simulink model "Autopilot_q_full_5may_new"  (R2020a)
settings: Solver=ode4  StartTime=0.0  StopTime=300  FixedStep=0.01  RelTol=1e-3
undefined symbols (not defined in the file or in its folder): Aero_cofficients, Atmosphere_pert, Atmospheric_model, Counter_sensor_model, Earth, error_global, flags_global, Guidance_Flags_global, INT_global, param_guidance, Payload_data, Plane_state_mode_finish_catcher_ftr_mode, Plane_state_mode_finish_catcher_fw_mode, Plane_state_mode_finish_catcher_q_mode, Plane_state_mode_finish_catcher_rtr_mode, Plane_state_store, propulsion_model, propulsion_model_int, Structural_data, Thrust_data_store, time_global, WGS84, Wind_data, Wind_model_int, Wind_pert_factor
libraries: simulink x33, aerolibactuator x15, cstblocks x3, aerolibatmos2 x2, aerolibfltsims x1, aerolibtransform2 x1, shared6dof x1
(part 9 of 10)

== matlab function Autopilot_q_full_5may_new/AUTOPILOT /Autopilot Fixed wing mode/Pitch controller/MATLAB Function3 ==
  data: a_z_d input; Plane_state input; aero_data input; structure_data input; alpha_d output; Thrust input; Wind_ned input; propulsion_data input; atmos_data input; data2 input; data3 input; data4 input; data5 input; data6 input; data7 input
function alpha_d = Autopilot(a_z_d,Plane_state, aero_data, structure_data, Thrust, Wind_ned,  propulsion_data, atmos_data, data2, data3, data4, data5, data6, data7)
%%
b1=propulsion_data(1); % b and d of vtol propellers
d1=propulsion_data(2);
b1_inv=1.0/b1;
%%
rho=atmos_data(4); % density
%%
Tzf1=Thrust(1);
Tzf2=Thrust(2);
Tzf3=Thrust(3);
Tzf4=Thrust(4);

Tzb5=Thrust(5);
Tzb6=Thrust(6);
Tzb7=Thrust(7);
Tzb8=Thrust(8);
Tx9=Thrust(9);
Tx10=Thrust(10);
delta_e=Thrust(11);
delta_a=Thrust(12);
delta_r=Thrust(13);


mass=structure_data(1,1);c=structure_data(1,2);b=structure_data(1,3);s=structure_data(1,4);
Ix=structure_data(1,5);Iy=structure_data(1,6);Iz=structure_data(1,7);
Ixy=structure_data(1,8);Ixz=structure_data(1,9);Iyz=structure_data(1,10);
x1=structure_data(1,11);x2=structure_data(1,12);y1=structure_data(1,13);y2=structure_data(1,14);
y3=structure_data(1,15);y4=structure_data(1,16);y5=structure_data(1,17);y6=structure_data(1,18);
y7=structure_data(1,19);y8=structure_data(1,20);y9=structure_data(1,21);y10=structure_data(1,22);
z1=structure_data(1,23);mb=structure_data(1,24);

T_by_W=2.0;

c0=Ix*Iz-Ixz^2;
c1=Ixz*(Ix-Iy+Iz)/c0;
c2=(Iz*(Iz-Iy)+Ixz^2)/c0;
c3=Iz/c0;
c4=Ixz/c0;
c5=(Iz-Ix)/c0;
c6=Ixz/Iy;
c7=((Ix-Iy)*Ix + Ixz^2)/c0;
c8=Ix/c0;
c3_inv=1/c3;
c8_inv=1/c8;

CLo =aero_data(1,1); CL_alpha=aero_data(1,2);CL_beta=aero_data(1,3); CL_delta_e=aero_data(1,4); CL_delta_a=aero_data(1,5); CL_delta_r=aero_data(1,6); CL_p=aero_data(1,7);CL_q=aero_data(1,8);CL_r=aero_data(1,9);

Cdo =aero_data(2,1); Cd_alpha=aero_data(2,2);Cd_beta=aero_data(2,3); Cd_delta_e=aero_data(2,4); Cd_delta_a=aero_data(2,5); Cd_delta_r=aero_data(2,6); Cd_p=aero_data(2,7);Cd_q=aero_data(2,8);Cd_r=aero_data(2,9);

CYo =aero_data(3,1); CY_alpha=aero_data(3,2);CY_beta=aero_data(3,3); CY_delta_e=aero_data(3,4); CY_delta_a=aero_data(3,5); CY_delta_r=aero_data(3,6); CY_p=aero_data(3,7);CY_q=aero_data(3,8);CY_r=aero_data(3,9);

Clo =aero_data(4,1); Cl_alpha=aero_data(4,2);Cl_beta=aero_data(4,3); Cl_delta_e=aero_data(4,4); Cl_delta_a=aero_data(4,5); Cl_delta_r=aero_data(4,6); Cl_p=aero_data(4,7);Cl_q=aero_data(4,8);Cl_r=aero_data(4,9);

Cmo =aero_data(5,1); Cm_alpha=aero_data(5,2);Cm_beta=aero_data(5,3); Cm_delta_e=aero_data(5,4); Cm_delta_a=aero_data(5,5); Cm_delta_r=aero_data(5,6); Cm_p=aero_data(5,7);Cm_q=aero_data(5,8);Cm_r=aero_data(5,9);

Cno =aero_data(6,1); Cn_alpha=aero_data(6,2);Cn_beta=aero_data(6,3); Cn_delta_e=aero_data(6,4); Cn_delta_a=aero_data(6,5); Cn_delta_r=aero_data(6,6); Cn_p=aero_data(6,7);Cn_q=aero_data(6,8);Cn_r=aero_data(6,9);
Cd_brake=0.0;brake=0.0;g=9.81;


u=Plane_state(1);
v=Plane_state(2);
w=Plane_state(3);
p=Plane_state(4);
q=Plane_state(5);
r=Plane_state(6);
phi=Plane_state(7);
theta=Plane_state(8);
psi=Plane_state(9);
X=Plane_state(10);
Y=Plane_state(11);
Z=Plane_state(12);


Tzf=Tzf2+Tzf3;
Tzb=Tzb6+Tzb7;
Tx=Tx9+Tx10;


R_v_v1=[cos(psi) sin(psi) 0; -sin(psi) cos(psi) 0; 0 0 1];
R_v1_v2=[cos(theta) 0 -sin(theta) ;0 1 0; sin(theta) 0 cos(theta)];
R_v2_b=[1 0 0;0 cos(phi) sin(phi) ;0 -sin(phi) cos(phi)];
R_v_b=R_v2_b*R_v1_v2*R_v_v1;



V_wind_bd=R_v_b*[Wind_ned(1);Wind_ned(2);Wind_ned(3)];

ppp = [u-V_wind_bd(1); v; w];
u_r=ppp(1);
v_r=ppp(2);
w_r=ppp(3);

V=sqrt(u_r^2+v_r^2+w_r^2);


if (u_r^2+v_r^2+w_r^2)<=0.01
    alpha=0;
else
    alpha=atan2( w_r, u_r);
end


if norm(u_r) < 10^-3  && norm(v_r) < 10^-3 && norm(w_r) < 10^-3
    beta=0;
else
    beta = asin(v_r/sqrt(u_r^2+v_r^2+w_r^2));
end



R_b_s=[cos(alpha) 0 sin(alpha) ;0 1 0; -sin(alpha) 0 cos(alpha)];
R_s_w=[cos(beta) sin(beta) 0; -sin(beta) cos(beta) 0; 0 0 1];
R_w_b=(R_b_s)'*(R_s_w)';


%u_dot_d=acc_d(1);
%v_dot_d=acc_d(2);
w_dot_d=a_z_d;



mg_b = R_v_b*[0 ;0; mass*g];
D=0.5*rho*V*V*s*(Cdo+Cd_alpha*abs(alpha)+Cd_delta_e*abs(delta_e)+ Cd_brake*abs(brake)) ;
D_b=R_w_b*[-D;0;0];

if V<0.1
    CL = CLo + CL_alpha*alpha + CL_delta_e*delta_e ;
else
    CL = CLo + CL_alpha*alpha + CL_delta_e*delta_e  + CL_q*q*c/(2*V) ;
end
L=0.5*rho*V*V*s*(CL);
%L_b = R_w_b*[0;0;-L];



fz=mass*w_dot_d;


alpha_d = (1.0/CL_alpha)*(((1.0/(-cos(alpha)*0.5*rho*V*V*s))*(fz - mg_b(3) - D_b(3))) - (CLo  + CL_delta_e*delta_e));


if (alpha_d > (10.0/57.3))
    alpha_d = (10.0/57.3);
end

if ((alpha_d) < (-5.0/57.3))
    
    alpha_d = -5.0/57.3;
end

== matlab function Autopilot_q_full_5may_new/AUTOPILOT /Autopilot Fixed wing mode/Roll controller/MATLAB Function1 ==
  data: t input; Thrust input; mass input; a_y_d input; phi_d output; aero_data input; structure_data input; Plane_state input; param_guidance input; Wind_ned input; propulsion_data input; atmos_data input; data2 input; data3 input; data5 input; data4 input; data6 input; data7 input
function phi_d  = fcn(t, Thrust, mass, a_y_d,aero_data, structure_data,Plane_state, param_guidance, Wind_ned, propulsion_data, atmos_data, data2, data3, data5, data4, data6, data7)
%%
b1=propulsion_data(1); % b and d of vtol propellers
d1=propulsion_data(2);
b1_inv=1.0/b1;
%%
rho=atmos_data(4); % density
%%
R_circ=param_guidance(1);
cruise_speed=param_guidance(2);

lmt_pos=param_guidance(3); lmt_vel=param_guidance(4);

Tzf1=Thrust(1);
Tzf2=Thrust(2);
Tzf3=Thrust(3);
Tzf4=Thrust(4);

Tzb5=Thrust(5);
Tzb6=Thrust(6);
Tzb7=Thrust(7);
Tzb8=Thrust(8);
Tx9=Thrust(9);
Tx10=Thrust(10);
delta_e=Thrust(11);
delta_a=Thrust(12);
delta_r=Thrust(13);

TT=abs(Tzf1+Tzf2+Tzf3+Tzf4+Tzb5+Tzb6+Tzb7+Tzb8);

mass=structure_data(1,1);c=structure_data(1,2);b=structure_data(1,3);s=structure_data(1,4);
% Ix=structure_data(1,5);Iy=structure_data(1,6);Iz=structure_data(1,7);
% Ixy=structure_data(1,8);Ixz=structure_data(1,9);Iyz=structure_data(1,10);
% x1=structure_data(1,11);x2=structure_data(1,12);y1=structure_data(1,13);y2=structure_data(1,14);
% y3=structure_data(1,15);y4=structure_data(1,16);y5=structure_data(1,17);y6=structure_data(1,18);
% y7=structure_data(1,19);y8=structure_data(1,20);y9=structure_data(1,21);y10=structure_data(1,22);
% z1=structure_data(1,23);mb=structure_data(1,24);
%
% T_by_W=2.0;

% c0=Ix*Iz-Ixz^2;
% c1=Ixz*(Ix-Iy+Iz)/c0;
% c2=(Iz*(Iz-Iy)+Ixz^2)/c0;
% c3=Iz/c0;
% c4=Ixz/c0;
% c5=(Iz-Ix)/c0;
% c6=Ixz/Iy;
% c7=((Ix-Iy)*Ix + Ixz^2)/c0;
% c8=Ix/c0;
% c3_inv=1/c3;
% c8_inv=1/c8;

CLo =aero_data(1,1); CL_alpha=aero_data(1,2);CL_beta=aero_data(1,3); CL_delta_e=aero_data(1,4); CL_delta_a=aero_data(1,5); CL_delta_r=aero_data(1,6); CL_p=aero_data(1,7);CL_q=aero_data(1,8);CL_r=aero_data(1,9);

% Cdo =aero_data(1,1); Cd_alpha=aero_data(1,2);Cd_beta=aero_data(1,3); Cd_delta_e=aero_data(1,4); Cd_delta_a=aero_data(1,5); Cd_delta_r=aero_data(1,6); Cd_p=aero_data(1,7);Cd_q=aero_data(1,8);Cd_r=aero_data(1,9);
%
% CYo =aero_data(1,1); CY_alpha=aero_data(1,2);CY_beta=aero_data(1,3); CY_delta_e=aero_data(1,4); CY_delta_a=aero_data(1,5); CY_delta_r=aero_data(1,6); CY_p=aero_data(1,7);CY_q=aero_data(1,8);CY_r=aero_data(1,9);
%
% Clo =aero_data(1,1); Cl_alpha=aero_data(1,2);Cl_beta=aero_data(1,3); Cl_delta_e=aero_data(1,4); Cl_delta_a=aero_data(1,5); Cl_delta_r=aero_data(1,6); Cl_p=aero_data(1,7);Cl_q=aero_data(1,8);Cl_r=aero_data(1,9);
%
% Cmo =aero_data(1,1); Cm_alpha=aero_data(1,2);Cm_beta=aero_data(1,3); Cm_delta_e=aero_data(1,4); Cm_delta_a=aero_data(1,5); Cm_delta_r=aero_data(1,6); Cm_p=aero_data(1,7);Cm_q=aero_data(1,8);Cm_r=aero_data(1,9);
%
% Cno =aero_data(1,1); Cn_alpha=aero_data(1,2);Cn_beta=aero_data(1,3); Cn_delta_e=aero_data(1,4); Cn_delta_a=aero_data(1,5); Cn_delta_r=aero_data(1,6); Cn_p=aero_data(1,7);Cn_q=aero_data(1,8);Cn_r=aero_data(1,9);

% Cd_brake=0.0;brake=0.0;g=9.81;
% b1=0.0007488;
% d1=0.00002828;
% b1_inv=1.0/b1;

u=Plane_state(1);
v=Plane_state(2);
w=Plane_state(3);
p=Plane_state(4);
q=Plane_state(5);
r=Plane_state(6);
phi=Plane_state(7);
theta=Plane_state(8);
psi=Plane_state(9);
% X=Plane_state(10);
% Y=Plane_state(11);
% Z=Plane_state(12);


R_v_v1=[cos(psi) sin(psi) 0; -sin(psi) cos(psi) 0; 0 0 1];
R_v1_v2=[cos(theta) 0 -sin(theta) ;0 1 0; sin(theta) 0 cos(theta)];
R_v2_b=[1 0 0;0 cos(phi) sin(phi) ;0 -sin(phi) cos(phi)];
R_v_b=R_v2_b*R_v1_v2*R_v_v1;



V_wind_bd=R_v_b*[Wind_ned(1);Wind_ned(2);Wind_ned(3)];

ppp = [u-V_wind_bd(1); v; w];
u_r=ppp(1);
v_r=ppp(2);
w_r=ppp(3);

V=sqrt(u_r^2+v_r^2+w_r^2);



if (u_r^2+v_r^2+w_r^2)<=0.01
    alpha=0;
else
    alpha=atan2( w_r, u_r);
end

if norm(u_r) < 10^-3  && norm(v_r) < 10^-3 && norm(w_r) < 10^-3
    beta=0;
else
    beta = asin(v_r/sqrt(u_r^2+v_r^2+w_r^2));
end



R_b_s=[cos(alpha) 0 sin(alpha) ;0 1 0; -sin(alpha) 0 cos(alpha)];
R_s_w=[cos(beta) sin(beta) 0; -sin(beta) cos(beta) 0; 0 0 1];
R_w_b=(R_b_s)'*(R_s_w)';

%
% mg_b = R_v_b*[0 ;0; mass*g];
% D=0.5*rho*V*V*s*(Cdo+Cd_alpha*abs(alpha)+Cd_delta_e*abs(delta_e)+ Cd_brake*abs(brake)) ;
% D_b=R_w_b*[-D;0;0];

if V<0.1
    CL = CLo + CL_alpha*alpha + CL_delta_e*delta_e ;
else
    CL = CLo + CL_alpha*alpha + CL_delta_e*delta_e  + CL_q*q*c/(2*V) ;
end

L=0.5*rho*V*V*s*(CL);



%phi_d=asin((mass/(TT-L_b(3)))*a_y_d);


if ((mass*cruise_speed^2/R_circ)/(abs(L))) > 0.5
    phi_d = sign(R_circ)*30/57.3;
else
    phi_d = asin((mass*cruise_speed^2/R_circ)/(abs(L)));
end
if L<(0.8*mass*9.81)
    phi_d=0.0;
end

if abs(phi_d)>30/57.3
    phi_d=sign(phi_d)*30/57.3;
end


end

== matlab function Autopilot_q_full_5may_new/AUTOPILOT /Autopilot Fixed wing mode/Roll controller/MATLAB Function2 ==
  data: angular_state input; phi_dot_d input; p_d output
function p_d  = fcn(angular_state,phi_dot_d)
p=angular_state(1);
q=angular_state(2);
r=angular_state(3);
phi=angular_state(4);
theta=angular_state(5);
psi=angular_state(6);
p_d= phi_dot_d - q*sin(phi)*tan(theta)-r*cos(phi)*tan(theta);

end

== matlab function Autopilot_q_full_5may_new/AUTOPILOT /Autopilot Transition mode/Reverse transition/Pitch Controller/MATLAB Function3 ==
  data: angular_state input; alpha_dot_d input; q_d output
function q_d  = fcn(angular_state,alpha_dot_d)

% p=angular_state(1);
% q=angular_state(2);
% r=angular_state(3);
% phi=angular_state(4);
% theta=angular_state(5);
% psi=angular_state(6);


		
	q_d=(alpha_dot_d );

	


end

== matlab function Autopilot_q_full_5may_new/AUTOPILOT /Autopilot Transition mode/Forward transition/Pitch Controller/alpha controller/MATLAB Function3 ==
  data: acc_d input; Plane_state input; aero_data input; structure_data input; alpha_d output; Thrust input; Wind_ned input; propulsion_data input; atmos_data input; data2 input; data3 input; data4 input; data5 input; data6 input; data7 input
function alpha_d = Autopilot(acc_d,Plane_state, aero_data, structure_data, Thrust, Wind_ned,  propulsion_data, atmos_data,  data2, data3, data4, data5, data6, data7)
%%
b1=propulsion_data(1); % b and d of vtol propellers
d1=propulsion_data(2);
b1_inv=1.0/b1;
%%
rho=atmos_data(4); % density
%%
Tzf1=Thrust(1);
Tzf2=Thrust(2);
Tzf3=Thrust(3);
Tzf4=Thrust(4);

Tzb5=Thrust(5);
Tzb6=Thrust(6);
Tzb7=Thrust(7);
Tzb8=Thrust(8);
Tx9=Thrust(9);
Tx10=Thrust(10);
delta_e=Thrust(11);
delta_a=Thrust(12);
delta_r=Thrust(13);


mass=structure_data(1,1);c=structure_data(1,2);b=structure_data(1,3);s=structure_data(1,4);
Ix=structure_data(1,5);Iy=structure_data(1,6);Iz=structure_data(1,7);
Ixy=structure_data(1,8);Ixz=structure_data(1,9);Iyz=structure_data(1,10);
x1=structure_data(1,11);x2=structure_data(1,12);y1=structure_data(1,13);y2=structure_data(1,14);
y3=structure_data(1,15);y4=structure_data(1,16);y5=structure_data(1,17);y6=structure_data(1,18);
y7=structure_data(1,19);y8=structure_data(1,20);y9=structure_data(1,21);y10=structure_data(1,22);
z1=structure_data(1,23);mb=structure_data(1,24);

T_by_W=2.0;

c0=Ix*Iz-Ixz^2; 
c1=Ixz*(Ix-Iy+Iz)/c0;    
c2=(Iz*(Iz-Iy)+Ixz^2)/c0;                                              
c3=Iz/c0;
c4=Ixz/c0;
c5=(Iz-Ix)/c0;
c6=Ixz/Iy;
c7=((Ix-Iy)*Ix + Ixz^2)/c0;
c8=Ix/c0;
c3_inv=1/c3;
c8_inv=1/c8;

CLo =aero_data(1,1); CL_alpha=aero_data(1,2);CL_beta=aero_data(1,3); CL_delta_e=aero_data(1,4); CL_delta_a=aero_data(1,5); CL_delta_r=aero_data(1,6); CL_p=aero_data(1,7);CL_q=aero_data(1,8);CL_r=aero_data(1,9);

Cdo =aero_data(2,1); Cd_alpha=aero_data(2,2);Cd_beta=aero_data(2,3); Cd_delta_e=aero_data(2,4); Cd_delta_a=aero_data(2,5); Cd_delta_r=aero_data(2,6); Cd_p=aero_data(2,7);Cd_q=aero_data(2,8);Cd_r=aero_data(2,9);

CYo =aero_data(3,1); CY_alpha=aero_data(3,2);CY_beta=aero_data(3,3); CY_delta_e=aero_data(3,4); CY_delta_a=aero_data(3,5); CY_delta_r=aero_data(3,6); CY_p=aero_data(3,7);CY_q=aero_data(3,8);CY_r=aero_data(3,9);

Clo =aero_data(4,1); Cl_alpha=aero_data(4,2);Cl_beta=aero_data(4,3); Cl_delta_e=aero_data(4,4); Cl_delta_a=aero_data(4,5); Cl_delta_r=aero_data(4,6); Cl_p=aero_data(4,7);Cl_q=aero_data(4,8);Cl_r=aero_data(4,9);

Cmo =aero_data(5,1); Cm_alpha=aero_data(5,2);Cm_beta=aero_data(5,3); Cm_delta_e=aero_data(5,4); Cm_delta_a=aero_data(5,5); Cm_delta_r=aero_data(5,6); Cm_p=aero_data(5,7);Cm_q=aero_data(5,8);Cm_r=aero_data(5,9);

Cno =aero_data(6,1); Cn_alpha=aero_data(6,2);Cn_beta=aero_data(6,3); Cn_delta_e=aero_data(6,4); Cn_delta_a=aero_data(6,5); Cn_delta_r=aero_data(6,6); Cn_p=aero_data(6,7);Cn_q=aero_data(6,8);Cn_r=aero_data(6,9);
Cd_brake=0.0;brake=0.0;g=9.81;


u=Plane_state(1);
v=Plane_state(2);
w=Plane_state(3);
p=Plane_state(4);
q=Plane_state(5);
r=Plane_state(6);
phi=Plane_state(7);
theta=Plane_state(8);
psi=Plane_state(9);
X=Plane_state(10);
Y=Plane_state(11);
Z=Plane_state(12);


        Tzf=Tzf2+Tzf3;
        Tzb=Tzb6+Tzb7;
        Tx=Tx9+Tx10;


R_v_v1=[cos(psi) sin(psi) 0; -sin(psi) cos(psi) 0; 0 0 1];
R_v1_v2=[cos(theta) 0 -sin(theta) ;0 1 0; sin(theta) 0 cos(theta)];
R_v2_b=[1 0 0;0 cos(phi) sin(phi) ;0 -sin(phi) cos(phi)];
R_v_b=R_v2_b*R_v1_v2*R_v_v1;



V_wind_bd=R_v_b*[Wind_ned(1);Wind_ned(2);Wind_ned(3)];

ppp = [u-V_wind_bd(1); v; w];
u_r=ppp(1);
v_r=ppp(2);
w_r=ppp(3);

V=sqrt(u_r^2+v_r^2+w_r^2);





if (u_r^2+v_r^2+w_r^2)<=0.01 
    alpha=0;
else
    alpha=atan2( w_r, u_r);
end

if norm(u_r) < 10^-3  && norm(v_r) < 10^-3 && norm(w_r) < 10^-3
    beta=0;
else
    beta = asin(v_r/sqrt(u_r^2+v_r^2+w_r^2));
end



R_b_s=[cos(alpha) 0 sin(alpha) ;0 1 0; -sin(alpha) 0 cos(alpha)]; 
R_s_w=[cos(beta) sin(beta) 0; -sin(beta) cos(beta) 0; 0 0 1];
R_w_b=(R_b_s)'*(R_s_w)';



u_dot_d=acc_d(1);
v_dot_d=acc_d(2);
w_dot_d=acc_d(3);


mg_b = R_v_b*[0 ;0; mass*g];
D=0.5*rho*V*V*s*(Cdo+Cd_alpha*abs(alpha)+Cd_delta_e*abs(delta_e)+ Cd_brake*abs(brake)) ;
D_b=R_w_b*[-D;0;0];

if V<0.1
    CL = CLo + CL_alpha*alpha + CL_delta_e*delta_e ;
else
    CL = CLo + CL_alpha*alpha + CL_delta_e*delta_e  + CL_q*q*c/(2*V) ;
end
L=0.5*rho*V*V*s*(CL);
L_b = R_w_b*[0;0;-L];

    
        fz=mass*w_dot_d;
    
        
        if (abs(cos(alpha)) >0.1)
        alpha_d = (1.0/CL_alpha)*(((1.0/(-cos(alpha)*0.5*rho*V*V*s))*(fz + (Tzf+Tzb) - mg_b(3) - D_b(3))) - (CLo  + CL_delta_e*delta_e)); 
        else
            alpha_d=3.0/57.3;
        end
       % alpha_d=5.0/57.3;
        
        if (alpha_d > (7.0/57.3))
        	alpha_d = (7.0/57.3);
        end

        if ((alpha_d) < (0.0/57.3))
        
        	alpha_d = 0.0/57.3;
        end

== matlab function Autopilot_q_full_5may_new/AUTOPILOT /Autopilot Transition mode/Forward transition/Pitch Controller/MATLAB Function3 ==
  data: alpha_dot_d input; angular_state input; q_d output
function q_d  = fcn(alpha_dot_d,angular_state)

% p=angular_state(1);
% q=angular_state(2);
% r=angular_state(3);
% phi=angular_state(4);
% theta=angular_state(5);
% psi=angular_state(6);


		
	q_d=(alpha_dot_d );

	


end

== matlab function Autopilot_q_full_5may_new/Wind_Model/Subsystem1/MATLAB Function ==
  data: u input; y output; Wind_model_int input; Z input
function y = fcn(u, Wind_model_int, Z)
y=u;
turb_50=Wind_model_int(8);
turb_50_600=Wind_model_int(9);
turb_600=Wind_model_int(10);

if ((turb_50 == 0) && (Z >=-50))
    y=0.0;  
end

if ((turb_50_600 == 0) && (Z >=-600) && (Z <=-50))
    y=0.0;  
end

if ((turb_600 == 0) && (Z <=-600))
    y=0.0;  
end

if Z>0.0
    y=0.0;
end
end

== matlab function Autopilot_q_full_5may_new/AUTOPILOT /Autopilot Transition mode/Reverse transition/Pitch Controller/MATLAB Function4 ==
  data: theta_dot_d input; angular_state input; q_d output
function q_d  = fcn(theta_dot_d,angular_state)

p=angular_state(1);
q=angular_state(2);
r=angular_state(3);
phi=angular_state(4);
theta=angular_state(5);
psi=angular_state(6);

if (abs(phi)>(pi/2.5))
		
	q_d=(theta_dot_d +r*sin(phi));
		
else
		
	q_d=(theta_dot_d +r*sin(phi))/cos(phi);
end

end

== matlab function Autopilot_q_full_5may_new/AUTOPILOT /Autopilot Transition mode/Reverse transition/Autopilot ==
  data: t input; p_dot_d input; q_dot_d input; r_dot_d input; acc_d input; Tzf1 output; Tzf2 output; Tzf3 output; Tzf4 output; Tzb5 output; Tzb6 output; Tzb7 output; Tzb8 output; Tx9 output; Tx10 output; delta_e output; delta_a output; delta_r output; Plane_state input; aero_data input; structure_data input; Thrust input; flags_global input; time_global input; stall_speed input; flags_global output; time_global output; Wind_ned input; propulsion_data input; atmos_data input; wind_pert_factor input; propulsion_pert_factor input; structure_pert_factor input; atmos_pert_factor input; aero_coff_pert_factor input; data7 input; data8 input; data9 input; data10 input; data11 input; data12 input
function [Tzf1,Tzf2,Tzf3,Tzf4,Tzb5,Tzb6,Tzb7,Tzb8,Tx9,Tx10,delta_e,delta_a,delta_r, flags_global,time_global] = Autopilot(t,p_dot_d,q_dot_d,r_dot_d,acc_d,Plane_state, aero_data, structure_data, Thrust,  flags_global,time_global, stall_speed, Wind_ned, propulsion_data, atmos_data, wind_pert_factor, propulsion_pert_factor, structure_pert_factor, atmos_pert_factor, aero_coff_pert_factor, data7, data8, data9, data10, data11, data12)
%%
b1=propulsion_data(1); % b and d of vtol propellers
d1=propulsion_data(2);
b1_inv=1.0/b1;
% b1 = b1*propulsion_pert_factor(1); % adding in perturbation in b and d
% d1 = d1*propulsion_pert_factor(2);
% b1_inv=1.0/b1;
%%
rho=atmos_data(4); % density
% rho = rho*atmos_pert_factor(4); % adding perturbation in density
%%
tf0=time_global(1);
tf1=time_global(2);
tf2=time_global(3);
tf3=time_global(4);
tf4=time_global(5);
tf5=time_global(6);
tf6=time_global(7);
tf7=time_global(8);
tf8=time_global(9);
%%
all_initial_check_ok=flags_global(1);
default_mode=flags_global(2);
quad_mode=flags_global(3);
Transition_mode=flags_global(4);
Fixed_wing_mode=flags_global(5);
fail_safe_mode=flags_global(6);
fail_safe_mode_hover=flags_global(7);
fail_safe_mode_land=flags_global(8);
fail_safe_mode_2=flags_global(9);
flag_initial_lift_off_hover = flags_global(10);
flag_vertical_takeoff = flags_global(11);
flag_hover_mode = flags_global(12);
flag_circle_mode =  flags_global(13);
flag_cruise_mode = flags_global(14);
flag_vertical_landing = flags_global(15);

one_time_initial_lift_off_hover = flags_global(16);
one_time_initial_vertical_takeoff = flags_global(17);
one_time_initial_hover_mode = flags_global(18);
one_time_initial_cruise_mode = flags_global(19);
one_time_initial_circle_mode = flags_global(20);
one_time_initial_vertical_landing = flags_global(21);

flag_brake_mode=flags_global(22);

flag_forward_transition=flags_global(23);
flag_reverse_transition=flags_global(24);

one_time_initial_flag_forward_transition = flags_global(25);
one_time_initial_flag_reverse_transition = flags_global(26);

%%

Tzf1=Thrust(1);
Tzf2=Thrust(2);
Tzf3=Thrust(3);
Tzf4=Thrust(4);

Tzb5=Thrust(5);
Tzb6=Thrust(6);
Tzb7=Thrust(7);
Tzb8=Thrust(8);
Tx9=Thrust(9);
Tx10=Thrust(10);
delta_e=Thrust(11);
delta_a=Thrust(12);
delta_r=Thrust(13);

%%
mass=structure_data(1,1);c=structure_data(1,2);b=structure_data(1,3);s=structure_data(1,4);
Ix=structure_data(1,5);Iy=structure_data(1,6);Iz=structure_data(1,7);
Ixy=structure_data(1,8);Ixz=structure_data(1,9);Iyz=structure_data(1,10);
x1=structure_data(1,11);x2=structure_data(1,12);y1=structure_data(1,13);y2=structure_data(1,14);
y3=structure_data(1,15);y4=structure_data(1,16);y5=structure_data(1,17);y6=structure_data(1,18);
y7=structure_data(1,19);y8=structure_data(1,20);y9=structure_data(1,21);y10=structure_data(1,22);
z9=structure_data(1,23);mb=structure_data(1,24);
z10=-z9;
 %%
% mass=mass*structure_pert_factor(1,1); % perturbation in structure data
% c=c*structure_pert_factor(1,2);b=b*structure_pert_factor(1,3);s=s*structure_pert_factor(1,4);
% Ix=Ix*structure_pert_factor(1,5);Iy=Iy*structure_pert_factor(1,6);Iz=Iz*structure_pert_factor(1,7);
% Ixy=Ixy*structure_pert_factor(1,8);Ixz=Ixz*structure_pert_factor(1,9);Iyz=Iyz*structure_pert_factor(1,10);
% x1=x1*structure_pert_factor(1,11);x2=x2*structure_pert_factor(1,12);
% y1=y1*structure_pert_factor(1,13);y2=y2*structure_pert_factor(1,14);y3=y3*structure_pert_factor(1,15);y4=y4*structure_pert_factor(1,16);
% y5=y5*structure_pert_factor(1,17);y6=y6*structure_pert_factor(1,18);y7=y7*structure_pert_factor(1,19);y8=y8*structure_pert_factor(1,20);
% y9=y9*structure_pert_factor(1,21);y10=y10*structure_pert_factor(1,22);
% z9=z9*structure_pert_factor(1,23);
% mb=mb*structure_pert_factor(1,24);
% z10=-z9;
% %%
T_by_W=2.0;
%%
c0=Ix*Iz-Ixz^2;
c1=Ixz*(Ix-Iy+Iz)/c0;
c2=(Iz*(Iz-Iy)+Ixz^2)/c0;
c3=Iz/c0;
c4=Ixz/c0;
c5=(Iz-Ix)/c0;
c6=Ixz/Iy;
c7=((Ix-Iy)*Ix + Ixz^2)/c0;
c8=Ix/c0;
c3_inv=1/c3;
c8_inv=1/c8;

%%
CLo =aero_data(1,1); CL_alpha=aero_data(1,2);CL_beta=aero_data(1,3); CL_delta_e=aero_data(1,4); CL_delta_a=aero_data(1,5); CL_delta_r=aero_data(1,6); CL_p=aero_data(1,7);CL_q=aero_data(1,8);CL_r=aero_data(1,9);

Cdo =aero_data(2,1); Cd_alpha=aero_data(2,2);Cd_beta=aero_data(2,3); Cd_delta_e=aero_data(2,4); Cd_delta_a=aero_data(2,5); Cd_delta_r=aero_data(2,6); Cd_p=aero_data(2,7);Cd_q=aero_data(2,8);Cd_r=aero_data(2,9);

CYo =aero_data(3,1); CY_alpha=aero_data(3,2);CY_beta=aero_data(3,3); CY_delta_e=aero_data(3,4); CY_delta_a=aero_data(3,5); CY_delta_r=aero_data(3,6); CY_p=aero_data(3,7);CY_q=aero_data(3,8);CY_r=aero_data(3,9);

Clo =aero_data(4,1); Cl_alpha=aero_data(4,2);Cl_beta=aero_data(4,3); Cl_delta_e=aero_data(4,4); Cl_delta_a=aero_data(4,5); Cl_delta_r=aero_data(4,6); Cl_p=aero_data(4,7);Cl_q=aero_data(4,8);Cl_r=aero_data(4,9);

Cmo =aero_data(5,1); Cm_alpha=aero_data(5,2);Cm_beta=aero_data(5,3); Cm_delta_e=aero_data(5,4); Cm_delta_a=aero_data(5,5); Cm_delta_r=aero_data(5,6); Cm_p=aero_data(5,7);Cm_q=aero_data(5,8);Cm_r=aero_data(5,9);

Cno =aero_data(6,1); Cn_alpha=aero_data(6,2);Cn_beta=aero_data(6,3); Cn_delta_e=aero_data(6,4); Cn_delta_a=aero_data(6,5); Cn_delta_r=aero_data(6,6); Cn_p=aero_data(6,7);Cn_q=aero_data(6,8);Cn_r=aero_data(6,9);

%% perturbation in Aero coffecients
% CLo =CLo*aero_coff_pert_factor(1,1); CL_alpha=CL_alpha*aero_coff_pert_factor(1,2);CL_beta=CL_beta*aero_coff_pert_factor(1,3); CL_delta_e=CL_delta_e*aero_coff_pert_factor(1,4); CL_delta_a=CL_delta_a*aero_coff_pert_factor(1,5); CL_delta_r=CL_delta_r*aero_coff_pert_factor(1,6); CL_p=CL_p*aero_coff_pert_factor(1,7);CL_q=CL_q*aero_coff_pert_factor(1,8);CL_r=CL_r*aero_coff_pert_factor(1,9);
% 
% Cdo =Cdo*aero_coff_pert_factor(2,1); Cd_alpha=Cd_alpha*aero_coff_pert_factor(2,2);Cd_beta=Cd_beta*aero_coff_pert_factor(2,3); Cd_delta_e=Cd_delta_e*aero_coff_pert_factor(2,4); Cd_delta_a=Cd_delta_a*aero_coff_pert_factor(2,5); Cd_delta_r=Cd_delta_r*aero_coff_pert_factor(2,6); Cd_p=Cd_p*aero_coff_pert_factor(2,7);Cd_q=Cd_q*aero_coff_pert_factor(2,8);Cd_r=Cd_r*aero_coff_pert_factor(2,9);
% 
% CYo =CYo*aero_coff_pert_factor(3,1); CY_alpha=CY_alpha*aero_coff_pert_factor(3,2);CY_beta=CY_beta*aero_coff_pert_factor(3,3); CY_delta_e=CY_delta_e*aero_coff_pert_factor(3,4); CY_delta_a=CY_delta_a*aero_coff_pert_factor(3,5); CY_delta_r=CY_delta_r*aero_coff_pert_factor(3,6); CY_p=CY_p*aero_coff_pert_factor(3,7);CY_q=CY_q*aero_coff_pert_factor(3,8);CY_r=CY_r*aero_coff_pert_factor(3,9);
% 
% Clo =Clo*aero_coff_pert_factor(4,1); Cl_alpha=Cl_alpha*aero_coff_pert_factor(4,2);Cl_beta=Cl_beta*aero_coff_pert_factor(4,3); Cl_delta_e=Cl_delta_e*aero_coff_pert_factor(4,4); Cl_delta_a=Cl_delta_a*aero_coff_pert_factor(4,5); Cl_delta_r=Cl_delta_r*aero_coff_pert_factor(4,6); Cl_p=Cl_p*aero_coff_pert_factor(4,7);Cl_q=Cl_q*aero_coff_pert_factor(4,8);Cl_r=Cl_r*aero_coff_pert_factor(4,9);
% 
% Cmo =Cmo*aero_coff_pert_factor(5,1); Cm_alpha=Cm_alpha*aero_coff_pert_factor(5,2);Cm_beta=Cm_beta*aero_coff_pert_factor(5,3); Cm_delta_e=Cm_delta_e*aero_coff_pert_factor(5,4); Cm_delta_a=Cm_delta_a*aero_coff_pert_factor(5,5); Cm_delta_r=Cm_delta_r*aero_coff_pert_factor(5,6); Cm_p=Cm_p*aero_coff_pert_factor(5,7);Cm_q=Cm_q*aero_coff_pert_factor(5,8);Cm_r=Cm_r*aero_coff_pert_factor(5,9);
% 
% Cno =Cno*aero_coff_pert_factor(6,1); Cn_alpha=Cn_alpha*aero_coff_pert_factor(6,2);Cn_beta=Cn_beta*aero_coff_pert_factor(6,3); Cn_delta_e=Cn_delta_e*aero_coff_pert_factor(6,4); Cn_delta_a=Cn_delta_a*aero_coff_pert_factor(6,5); Cn_delta_r=Cn_delta_r*aero_coff_pert_factor(6,6); Cn_p=Cn_p*aero_coff_pert_factor(6,7);Cn_q=Cn_q*aero_coff_pert_factor(6,8);Cn_r=Cn_r*aero_coff_pert_factor(6,9);
%%
Cd_brake=0.0;brake=0.0;g=9.81;
%%
u=Plane_state(1);
v=Plane_state(2);
w=Plane_state(3);
p=Plane_state(4);
q=Plane_state(5);
r=Plane_state(6);
phi=Plane_state(7);
theta=Plane_state(8);
psi=Plane_state(9);
X=Plane_state(10);
Y=Plane_state(11);
Z=Plane_state(12);
%%
Tzf=Tzf2+Tzf3;
Tzb=Tzb6+Tzb7;
Tx=Tx9+Tx10;
%%

R_v_v1=[cos(psi) sin(psi) 0; -sin(psi) cos(psi) 0; 0 0 1];
R_v1_v2=[cos(theta) 0 -sin(theta) ;0 1 0; sin(theta) 0 cos(theta)];
R_v2_b=[1 0 0;0 cos(phi) sin(phi) ;0 -sin(phi) cos(phi)];
R_v_b=R_v2_b*R_v1_v2*R_v_v1;

%%
% 
% Wind_ned(1)=Wind_ned(1)*wind_pert_factor(1);% adding perturbation to wind components
% Wind_ned(2)=Wind_ned(2)*wind_pert_factor(2);
% Wind_ned(3)=Wind_ned(3)*wind_pert_factor(3);

V_wind_bd=R_v_b*[Wind_ned(1);Wind_ned(2);Wind_ned(3)];

ppp = [u-V_wind_bd(1); v; w];
u_r=ppp(1);
v_r=ppp(2);
w_r=ppp(3);

V=sqrt(u_r^2+v_r^2+w_r^2);

%%

if (u_r^2+v_r^2+w_r^2)<=0.01
    alpha=0;
else
    alpha=atan2( w_r, u_r);
end


if norm(u_r) < 10^-3  && norm(v_r) < 10^-3 && norm(w_r) < 10^-3
    beta=0;
else
    beta = asin(v_r/sqrt(u_r^2+v_r^2+w_r^2));
end

%%

R_b_s=[cos(alpha) 0 sin(alpha) ;0 1 0; -sin(alpha) 0 cos(alpha)];
R_s_w=[cos(beta) sin(beta) 0; -sin(beta) cos(beta) 0; 0 0 1];
R_w_b=(R_b_s)'*(R_s_w)';
%%
u_dot_d=acc_d(1);
v_dot_d=acc_d(2);
w_dot_d=acc_d(3);
%%
mg_b = R_v_b*[0 ;0; mass*g];
D=0.5*rho*V*V*s*(Cdo+Cd_alpha*abs(alpha)+Cd_delta_e*abs(delta_e)+ Cd_brake*abs(brake)) ;
D_b=R_w_b*[-D;0;0];

if V<0.1
    CL = CLo + CL_alpha*alpha + CL_delta_e*delta_e ;
else
    CL = CLo + CL_alpha*alpha + CL_delta_e*delta_e  + CL_q*q*c/(2*V) ;
end
L=0.5*rho*V*V*s*(CL);
L_b = R_w_b*[0;0;-L];
if abs(V)<0.1
    CY=CYo + CY_delta_r*delta_r + CY_beta*beta;
else
    CY=CYo + CY_delta_r*delta_r + CY_beta*beta + CY_r*r*b/(2*V);
end
FY=0.5*rho*V*V*s*(CY);
%%
w1=(mass*0.99*g- 0.5*rho*V*V*s*CL)/(0.99*mass*g);
w2=1-w1;
w3=1;
if w1<0.0
    w1=0.0;
    w2=1;
    w3=1;
end

if (u_r<(stall_speed)/2)
    w1=1.0;
    w2=0.0;
    w3=1.0;
end

%%


% if w1<0.05
%
% w1=0.0;
% w2=1.0;
% w3=1.0;
%
%
% Fixed_wing_mode=1;
% Transition_mode=0;
%
% tf4=t;
% end



l_aero=0.5*rho*V^2*s*b*( Clo + Cl_delta_a*delta_a +Cl_delta_r*delta_r +Cl_beta*beta )+0.5*rho*V*s*b*(Cl_p*p*b/2+Cl_r*r*b/2);
m_aero=0.5*rho*V^2*s*c*( Cmo + Cm_alpha*alpha + Cm_delta_e*delta_e)+0.5*rho*V*s*c*Cm_q*q*c/2;
n_aero=0.5*rho*V^2*s*b*( Cno + Cn_delta_a*delta_a +Cn_delta_r*delta_r +Cn_beta*beta )+0.5*rho*V*s*b*(Cn_r*r*b/2+ Cn_p*p*b/2);


l=l_aero...
    + (d1*Tx9*b1_inv) + (d1*Tx10*b1_inv)...
    + (- Tzf2*y2*cos(mb) - Tzf3*y3*cos(mb)   - Tzb6*y6*cos(mb) - Tzb7*y7*cos(mb))...
    + (- Tzf1*y1*cos(mb) - Tzf4*y4*cos(mb)   - Tzb5*y5*cos(mb) - Tzb8*y8*cos(mb));


m=m_aero ...
    + Tx9*z9 + Tx10*z10...
    + Tzf*x1*cos(mb) + Tzb*x2*cos(mb)...
    + d1*Tzf2*b1_inv*sin(mb) - d1*Tzf3*b1_inv*sin(mb) - d1*Tzb6*b1_inv*sin(mb) + d1*Tzb7*b1_inv*sin(mb)...
    + d1*Tzf1*b1_inv*sin(mb) - d1*Tzf4*b1_inv*sin(mb) - d1*Tzb5*b1_inv*sin(mb) + d1*Tzb8*b1_inv*sin(mb);

n=n_aero ...
    - Tx9*y9 - Tx10*y10 ...
    + (Tzf2*x1*sin(mb) - Tzf3*x1*sin(mb) +  Tzb6*x2*sin(mb) - Tzb7*x2*sin(mb))...
    + (Tzf1*x1*sin(mb) - Tzf4*x1*sin(mb) +  Tzb5*x2*sin(mb) - Tzb8*x2*sin(mb))...
    + (- d1*Tzf2*b1_inv*cos(mb) + d1*Tzf3*b1_inv*cos(mb)  + d1*Tzb6*b1_inv*cos(mb)  - d1*Tzb7*b1_inv*cos(mb))...
    + (- d1*Tzf1*b1_inv*cos(mb) + d1*Tzf4*b1_inv*cos(mb)  + d1*Tzb5*b1_inv*cos(mb)  - d1*Tzb8*b1_inv*cos(mb)) ;



% 	fx = Tx9 + Tx10 + D_b(1)+ mg_b(1)+L_b(1);
% 	%%%%%%%%%%%%%%%%%%%%%%%%%%%%%%%%%%%%%%%%%%%%%%%%%%%%%%%%%%%%%%%%%%%%%%%%%%%
% 	fy = (Tzf2*sin(mb) - Tzf3*sin(mb) + Tzb6*sin(mb) - Tzb7*sin(mb)) + D_b(2) + mg_b(2) + FY + L_b(2);
% 	%%%%%%%%%%%%%%%%%%%%%%%%%%%%%%%%%%%%%%%%%%%%%%%%%%%%%%%%%%%%%%%%%%%%%%%%%%%
% 	fz = -Tzf*cos(mb) - Tzb*cos(mb) + mg_b(3)+D_b(3)+L_b(3);
%
%
fx=mass*u_dot_d;
fy=mass*v_dot_d;
fz=mass*w_dot_d;

tam=[-b1*y2,-b1*y3,-b1*y6,-b1*y7; b1*x1,b1*x1,b1*x2,b1*x2; -d1,d1,d1,-d1; -b1,-b1,-b1,-b1];
tbm=zeros(4,1);

tbm(1)=(((p_dot_d - c1*p*q + c2*(q*r) -c4*n)*c3_inv) - l_aero)*w1;%//(((p_dot_d - c1*p*q + c2*(q*r) -c4*n)/c3) - l_aero)*w1*3/8
tbm(2)=(((q_dot_d - c5*p*r + c6*(p*p-r*r))*Iy) - m_aero)*w1;%//(((q_dot_d - c5*p*r + c6*(p*p-r*r))*Iy) - m_aero)*w1/2
tbm(3)=(((r_dot_d - c7*p*q + c1*(q*r) -c4*l)*c8_inv) - n_aero)*w1;%//(((r_dot_d - c7*p*q + c1*(q*r) -c4*l)/c8) - n_aero)*w1/2
tbm(4)=(fz - mg_b(3) - D_b(3) -L_b(3))*w3;%//(mass*w_dot_d - mg_b(3) - D_b(3) -L_b(3))/2

omega_velocity=inv(tam)*tbm;

for i=1:4
    if omega_velocity(i)<0.0
        omega_velocity(i)=0.0;
    end
end
omega_2=sqrt(omega_velocity(1));
omega_3=sqrt(omega_velocity(2));
omega_6=sqrt(omega_velocity(3));
omega_7=sqrt(omega_velocity(4));


Tzf2=b1*omega_2^2;

Tzf3=b1*omega_3^2;

Tzb6=b1*omega_6^2;

Tzb7=b1*omega_7^2;



% tam=[-b1*y1,-b1*y4,-b1*y5,-b1*y8; b1*x1,b1*x1,b1*x2,b1*x2; -d1,d1,d1,-d1; -b1,-b1,-b1,-b1];
% tbm=zeros(4,1);
%
% tbm(1)=(((p_dot_d - c1*p*q + c2*(q*r) -c4*n)*c3_inv) - l_aero)*w1;%//(((p_dot_d - c1*p*q + c2*(q*r) -c4*n)/c3) - l_aero)*w1*3/8
% tbm(2)=(((q_dot_d - c5*p*r + c6*(p*p-r*r))*Iy) - m_aero)*w1;%//(((q_dot_d - c5*p*r + c6*(p*p-r*r))*Iy) - m_aero)*w1/2
% tbm(3)=(((r_dot_d - c7*p*q + c1*(q*r) -c4*l)*c8_inv) - n_aero)*w1;%//(((r_dot_d - c7*p*q + c1*(q*r) -c4*l)/c8) - n_aero)*w1/2
% tbm(4)=(fz - mg_b(3) - D_b(3) -L_b(3))*w3;%//(mass*w_dot_d - mg_b(3) - D_b(3) -L_b(3))/2
%
% omega_velocity=inv(tam)*tbm;
%
% for i=1:4
%     if omega_velocity(i)<0.0
%         omega_velocity(i)=0.0;
%     end
% end
% omega_1=sqrt(omega_velocity(1));
% omega_4=sqrt(omega_velocity(2));
% omega_5=sqrt(omega_velocity(3));
% omega_8=sqrt(omega_velocity(4));
%
%
% Tzf1=b1*omega_1^2;
%
% Tzf4=b1*omega_4^2;
%
% Tzb5=b1*omega_5^2;
%
% Tzb8=b1*omega_8^2;
%

Tzf1=0.0;
Tzf4=0.0;
Tzb5=0.0;
Tzb8=0.0;
Tx10=0.0;

Tx9= fx - (D_b(1)+ mg_b(1)+L_b(1));

Tx9=0.0;

Tzf=Tzf2+Tzf3 + Tzf1 + Tzf4;
Tzb=Tzb6+Tzb7 + Tzb5 + Tzb8;
Tx=Tx9+Tx10;


if (u_r<(stall_speed)/2)
    delta_e=0.0;
    delta_r=0.0;
    delta_a=0.0;
else
    delta_e = (1.0/Cm_delta_e)*(((w2*Iy/(0.5*rho*V*V*s*c))*(q_dot_d - c5*p*r + c6*(p*p-r*r) -((0.0*1.0/Iy)*(Tzf*x1 + Tzb*x2 + Tx9*z9)) )) - (Cmo + Cm_alpha*alpha + (Cm_q*q*c/(2.0*V)))) ;
    delta_a =  (((w2/(0.5*rho*V*V*s*b*c3))*(p_dot_d - c1*p*q + c2*q*r - c4*n))  - (Clo + Cl_beta*beta + Cl_delta_r*delta_r + Cl_r*r*b/(2.0*V) +(Cl_p*p*b/(2.0*V))))/(Cl_delta_a);
    delta_r =  (((w2/(0.5*rho*V*V*s*b*c8))*(r_dot_d - c7*p*q + c1*q*r - c4*l))  - (Cno + Cn_beta*beta + Cn_delta_a*delta_a + Cn_r*r*b/(2.0*V) +(Cn_p*p*b/(2.0*V))))/(Cn_delta_r);
end



if abs(delta_e)>(20.0/57.3)
    delta_e=sign(delta_e)*(20.0/57.3);
end

if abs(delta_a)>(20.0/57.3)
    delta_a=sign(delta_a)*(20.0/57.3);
end

if abs(delta_r)>(20.0/57.3)
    delta_r=sign(delta_r)*(20.0/57.3);
end





if (Tzf > (T_by_W*mass*g)/2.0)
    
    Tzf=(T_by_W*mass*g)/2.0;
end



if(Tzf<= 0.0)
    
    Tzf=0.0;
end

if(Tzb> (T_by_W*mass*g)/2.0)
    
    Tzb=(T_by_W*mass*g)/2.0;
end
if(Tzb<= 0.0)
    
    Tzb=0.0;
end


if(Tzf2<=0.0)
    
    Tzf2=0.0;
end
if(Tzf3<= 0.0)
    
    Tzf3=0.0;
end
if(Tzb6<= 0.0)
    
    Tzb6=0.0;
end
if(Tzb7<=0.0)
    
    Tzb7=0.0;
end
if(Tzf1<=0.0)
    
    Tzf1=0.0;
end
if(Tzf4<= 0.0)
    
    Tzf4=0.0;
end
if(Tzb5<= 0.0)
    
    Tzb5=0.0;
end
if(Tzb8<=0.0)
    
    Tzb8=0.0;
end

if(Tx>120.0)
    
    Tx=120.0;
end

if(Tx< 0.0)
    Tx=0.0;
end

if((Tx9)>120.0)
    Tx9=120.0;
end

if(Tx9 < 0.0)
    Tx9=0.0;
end

if((Tx10)>120.0)
    Tx10=120.0;
end

if(Tx10 < 0.0)
    Tx10=0.0;
end

if(Tzf2>(T_by_W*mass*g)/4.0)
    
    Tzf2 =(T_by_W*mass*g)/4.0;
end

if(Tzf3>=(T_by_W*mass*g)/4.0)
    
    Tzf3 =(T_by_W*mass*g)/4.0;
end

if(Tzb6>=(T_by_W*mass*g)/4.0)
    
    Tzb6 =(T_by_W*mass*g)/4.0;
end

if(Tzb7>=(T_by_W*mass*g)/4.0)
    
    Tzb7 =(T_by_W*mass*g)/4.0;
end


if(Tzf1>(T_by_W*mass*g)/4.0)
    
    Tzf1 =(T_by_W*mass*g)/4.0;
end

if(Tzf4>=(T_by_W*mass*g)/4.0)
    
    Tzf4 =(T_by_W*mass*g)/4.0;
end

if(Tzb5>=(T_by_W*mass*g)/4.0)
    
    Tzb5 =(T_by_W*mass*g)/4.0;
end

if(Tzb8>=(T_by_W*mass*g)/4.0)
    
    Tzb8 =(T_by_W*mass*g)/4.0;
end



flags_global(1)=all_initial_check_ok;
flags_global(2)=default_mode;

flags_global(3)=quad_mode;
flags_global(4)=Transition_mode;
flags_global(5)=Fixed_wing_mode;

flags_global(6)=fail_safe_mode;
flags_global(7)=fail_safe_mode_hover;
flags_global(8)=fail_safe_mode_land;
flags_global(9)=fail_safe_mode_2;


flags_global(10)=flag_initial_lift_off_hover;
flags_global(11)=flag_vertical_takeoff;
flags_global(12)=flag_hover_mode;

flags_global(13)=flag_circle_mode;
flags_global(14)=flag_cruise_mode;

flags_global(15)=flag_vertical_landing;

flags_global(16)=one_time_initial_lift_off_hover;
flags_global(17)=one_time_initial_vertical_takeoff;
flags_global(18)=one_time_initial_hover_mode;
flags_global(19)=one_time_initial_cruise_mode;

flags_global(20)=one_time_initial_circle_mode;
flags_global(21)=one_time_initial_vertical_landing;
flags_global(22)=flag_brake_mode;

flags_global(23)=flag_forward_transition;
flags_global(24)=flag_reverse_transition;
flags_global(25)=one_time_initial_flag_forward_transition;
flags_global(26)=one_time_initial_flag_reverse_transition ;



time_global(1)=tf0;
time_global(2)=tf1;
time_global(3)=tf2;
time_global(4)=tf3;
time_global(5)=tf4;
time_global(6)=tf5;
time_global(7)=tf6;
time_global(8)=tf7;
time_global(9)=tf8;






end

== matlab function Autopilot_q_full_5may_new/AUTOPILOT /Autopilot Transition mode/Reverse transition/MATLAB Function7 ==
  data: v_dot_d output; Plane_state input; data input; acc_d input; u_dot_d output; w_dot_d output; V output
function [v_dot_d,u_dot_d,w_dot_d,V] = fcn(Plane_state, data, acc_d)

u=Plane_state(1);
v=Plane_state(2);
w=Plane_state(3);



V=sqrt(u^2 + v^2 + w^2);

u_dot_d=acc_d(1);
v_dot_d=acc_d(2);
w_dot_d=acc_d(3);

end

== matlab function Autopilot_q_full_5may_new/AUTOPILOT /Autopilot Transition mode/Reverse transition/Trim setting/MATLAB Function ==
  data: aero_data input; structure_data input; V_trim input; alpha_trim output; beta_trim output; delta_e_trim output; delta_a_trim output; delta_r_trim output; Tx_trim output; stall_speed output; propulsion_data input; atmos_data input
function [alpha_trim,beta_trim,delta_e_trim,delta_a_trim,delta_r_trim,Tx_trim,stall_speed]= Autopilot(aero_data,structure_data,V_trim,propulsion_data, atmos_data)
b1=propulsion_data(1); % b and d of vtol propellers
d1=propulsion_data(2);
b1_inv=1.0/b1;
%%
rho=atmos_data(4); % density
%%
V=V_trim;
mass=structure_data(1,1);s=structure_data(1,4);

CLo =aero_data(1,1); CL_alpha=aero_data(1,2);CL_beta=aero_data(1,3); CL_delta_e=aero_data(1,4); CL_delta_a=aero_data(1,5); CL_delta_r=aero_data(1,6); CL_p=aero_data(1,7);CL_q=aero_data(1,8);CL_r=aero_data(1,9);

Cdo =aero_data(2,1); Cd_alpha=aero_data(2,2);Cd_beta=aero_data(2,3); Cd_delta_e=aero_data(2,4); Cd_delta_a=aero_data(2,5); Cd_delta_r=aero_data(2,6); Cd_p=aero_data(2,7);Cd_q=aero_data(2,8);Cd_r=aero_data(2,9);

CYo =aero_data(3,1); CY_alpha=aero_data(3,2);CY_beta=aero_data(3,3); CY_delta_e=aero_data(3,4); CY_delta_a=aero_data(3,5); CY_delta_r=aero_data(3,6); CY_p=aero_data(3,7);CY_q=aero_data(3,8);CY_r=aero_data(3,9);

Clo =aero_data(4,1); Cl_alpha=aero_data(4,2);Cl_beta=aero_data(4,3); Cl_delta_e=aero_data(4,4); Cl_delta_a=aero_data(4,5); Cl_delta_r=aero_data(4,6); Cl_p=aero_data(4,7);Cl_q=aero_data(4,8);Cl_r=aero_data(4,9);

Cmo =aero_data(5,1); Cm_alpha=aero_data(5,2);Cm_beta=aero_data(5,3); Cm_delta_e=aero_data(5,4); Cm_delta_a=aero_data(5,5); Cm_delta_r=aero_data(5,6); Cm_p=aero_data(5,7);Cm_q=aero_data(5,8);Cm_r=aero_data(5,9);

Cno =aero_data(6,1); Cn_alpha=aero_data(6,2);Cn_beta=aero_data(6,3); Cn_delta_e=aero_data(6,4); Cn_delta_a=aero_data(6,5); Cn_delta_r=aero_data(6,6); Cn_p=aero_data(6,7);Cn_q=aero_data(6,8);Cn_r=aero_data(6,9);



g=9.81;



tb=[(mass*g/(0.5*rho*V*V*s)) - CLo;-Cmo];
ta=[CL_alpha,CL_delta_e;Cm_alpha,Cm_delta_e];

trim_set_long = inv(ta)*tb;

alpha_trim = trim_set_long(1);
delta_e_trim = trim_set_long(2);

% CYo + CY_beta*beta + CY_delta_a*delta_a + CY_delta_r*delta_r;
% Clo + Cl_beta*beta + Cl_delta_a*delta_a + Cl_delta_r*delta_r;
% Cno + Cn_beta*beta + Cn_delta_a*delta_a + Cn_delta_r*delta_r;

tb1=[-CYo;-Clo;-Cno];
ta1=[CY_beta,CY_delta_a,CY_delta_r;Cl_beta,Cl_delta_a,Cl_delta_r;Cn_beta,Cn_delta_a,Cn_delta_r];

trim_set_lat=inv(ta1)*tb1;

beta_trim = trim_set_lat(1);
delta_a_trim = trim_set_lat(2);
delta_r_trim = trim_set_lat(3);


% drag = 1/2 *rho *V*V*s*( Cdo + Cd_alpha*alpha + Cd_delta_e*delta_e );
Tx_trim =  0.5*rho*V*V*s*( Cdo + Cd_alpha*alpha_trim + Cd_delta_e*delta_e_trim );

stall_speed=sqrt((mass*g)/(0.5*1.225*s*(CLo+CL_alpha*(12.0/57.3))));

== matlab function Autopilot_q_full_5may_new/AUTOPILOT /Autopilot Transition mode/Reverse transition/Pitch Controller/alpha controller/MATLAB Function3 ==
  data: acc_d input; Plane_state input; aero_data input; structure_data input; alpha_d output; Thrust input; Wind_ned input; propulsion_data input; atmos_data input; data2 input; data3 input; data4 input; data5 input; data6 input; data7 input
function alpha_d = Autopilot(acc_d,Plane_state, aero_data, structure_data, Thrust, Wind_ned, propulsion_data, atmos_data, data2, data3, data4, data5, data6, data7)
%%
b1=propulsion_data(1); % b and d of vtol propellers
d1=propulsion_data(2);
b1_inv=1.0/b1;
%%
rho=atmos_data(4); % density
%%
Tzf1=Thrust(1);
Tzf2=Thrust(2);
Tzf3=Thrust(3);
Tzf4=Thrust(4);

Tzb5=Thrust(5);
Tzb6=Thrust(6);
Tzb7=Thrust(7);
Tzb8=Thrust(8);
Tx9=Thrust(9);
Tx10=Thrust(10);
delta_e=Thrust(11);
delta_a=Thrust(12);
delta_r=Thrust(13);


mass=structure_data(1,1);c=structure_data(1,2);b=structure_data(1,3);s=structure_data(1,4);
Ix=structure_data(1,5);Iy=structure_data(1,6);Iz=structure_data(1,7);
Ixy=structure_data(1,8);Ixz=structure_data(1,9);Iyz=structure_data(1,10);
x1=structure_data(1,11);x2=structure_data(1,12);y1=structure_data(1,13);y2=structure_data(1,14);
y3=structure_data(1,15);y4=structure_data(1,16);y5=structure_data(1,17);y6=structure_data(1,18);
y7=structure_data(1,19);y8=structure_data(1,20);y9=structure_data(1,21);y10=structure_data(1,22);
z1=structure_data(1,23);mb=structure_data(1,24);

T_by_W=2.0;

c0=Ix*Iz-Ixz^2;
c1=Ixz*(Ix-Iy+Iz)/c0;
c2=(Iz*(Iz-Iy)+Ixz^2)/c0;
c3=Iz/c0;
c4=Ixz/c0;
c5=(Iz-Ix)/c0;
c6=Ixz/Iy;
c7=((Ix-Iy)*Ix + Ixz^2)/c0;
c8=Ix/c0;
c3_inv=1/c3;
c8_inv=1/c8;

CLo =aero_data(1,1); CL_alpha=aero_data(1,2);CL_beta=aero_data(1,3); CL_delta_e=aero_data(1,4); CL_delta_a=aero_data(1,5); CL_delta_r=aero_data(1,6); CL_p=aero_data(1,7);CL_q=aero_data(1,8);CL_r=aero_data(1,9);

Cdo =aero_data(2,1); Cd_alpha=aero_data(2,2);Cd_beta=aero_data(2,3); Cd_delta_e=aero_data(2,4); Cd_delta_a=aero_data(2,5); Cd_delta_r=aero_data(2,6); Cd_p=aero_data(2,7);Cd_q=aero_data(2,8);Cd_r=aero_data(2,9);

CYo =aero_data(3,1); CY_alpha=aero_data(3,2);CY_beta=aero_data(3,3); CY_delta_e=aero_data(3,4); CY_delta_a=aero_data(3,5); CY_delta_r=aero_data(3,6); CY_p=aero_data(3,7);CY_q=aero_data(3,8);CY_r=aero_data(3,9);

Clo =aero_data(4,1); Cl_alpha=aero_data(4,2);Cl_beta=aero_data(4,3); Cl_delta_e=aero_data(4,4); Cl_delta_a=aero_data(4,5); Cl_delta_r=aero_data(4,6); Cl_p=aero_data(4,7);Cl_q=aero_data(4,8);Cl_r=aero_data(4,9);

Cmo =aero_data(5,1); Cm_alpha=aero_data(5,2);Cm_beta=aero_data(5,3); Cm_delta_e=aero_data(5,4); Cm_delta_a=aero_data(5,5); Cm_delta_r=aero_data(5,6); Cm_p=aero_data(5,7);Cm_q=aero_data(5,8);Cm_r=aero_data(5,9);

Cno =aero_data(6,1); Cn_alpha=aero_data(6,2);Cn_beta=aero_data(6,3); Cn_delta_e=aero_data(6,4); Cn_delta_a=aero_data(6,5); Cn_delta_r=aero_data(6,6); Cn_p=aero_data(6,7);Cn_q=aero_data(6,8);Cn_r=aero_data(6,9);
Cd_brake=0.0;brake=0.0;g=9.81;

u=Plane_state(1);
v=Plane_state(2);
w=Plane_state(3);
p=Plane_state(4);
q=Plane_state(5);
r=Plane_state(6);
phi=Plane_state(7);
theta=Plane_state(8);
psi=Plane_state(9);
X=Plane_state(10);
Y=Plane_state(11);
Z=Plane_state(12);


Tzf=Tzf2+Tzf3;
Tzb=Tzb6+Tzb7;
Tx=Tx9+Tx10;


R_v_v1=[cos(psi) sin(psi) 0; -sin(psi) cos(psi) 0; 0 0 1];
R_v1_v2=[cos(theta) 0 -sin(theta) ;0 1 0; sin(theta) 0 cos(theta)];
R_v2_b=[1 0 0;0 cos(phi) sin(phi) ;0 -sin(phi) cos(phi)];
R_v_b=R_v2_b*R_v1_v2*R_v_v1;




V_wind_bd=R_v_b*[Wind_ned(1);Wind_ned(2);Wind_ned(3)];

ppp = [u-V_wind_bd(1); v; w];
u_r=ppp(1);
v_r=ppp(2);
w_r=ppp(3);

V=sqrt(u_r^2+v_r^2+w_r^2);



if (u_r^2+v_r^2+w_r^2)<=0.01
    alpha=0;
else
    alpha=atan2( w_r, u_r);
end

if norm(u_r) < 10^-3  && norm(v_r) < 10^-3 && norm(w_r) < 10^-3
    beta=0;
else
    beta = asin(v_r/sqrt(u_r^2+v_r^2+w_r^2));
end



R_b_s=[cos(alpha) 0 sin(alpha) ;0 1 0; -sin(alpha) 0 cos(alpha)];
R_s_w=[cos(beta) sin(beta) 0; -sin(beta) cos(beta) 0; 0 0 1];
R_w_b=(R_b_s)'*(R_s_w)';



u_dot_d=acc_d(1);
v_dot_d=acc_d(2);
w_dot_d=acc_d(3);


mg_b = R_v_b*[0 ;0; mass*g];
D=0.5*rho*V*V*s*(Cdo+Cd_alpha*abs(alpha)+Cd_delta_e*abs(delta_e)+ Cd_brake*abs(brake)) ;
D_b=R_w_b*[-D;0;0];

if V<0.1
    CL = CLo + CL_alpha*alpha + CL_delta_e*delta_e ;
else
    CL = CLo + CL_alpha*alpha + CL_delta_e*delta_e  + CL_q*q*c/(2*V) ;
end
L=0.5*rho*V*V*s*(CL);
L_b = R_w_b*[0;0;-L];


fz=mass*w_dot_d;


if (abs(cos(alpha)) >0.1)
    alpha_d = (1.0/CL_alpha)*(((1.0/(-cos(alpha)*0.5*rho*V*V*s))*(fz + (Tzf+Tzb) - mg_b(3) - D_b(3))) - (CLo  + CL_delta_e*delta_e));
else
    alpha_d=10.0/57.3;
end
% alpha_d=5.0/57.3;

if (alpha_d > (10.0/57.3))
    alpha_d = (10.0/57.3);
end

if ((alpha_d) < (0.0/57.3))
    
    alpha_d = 0.0/57.3;
end

== matlab function Autopilot_q_full_5may_new/AUTOPILOT /Autopilot Transition mode/Reverse transition/Roll controller/MATLAB Function1 ==
  data: t input; Thrust input; mass input; a_y_d input; phi_d output; aero_data input; structure_data input; Plane_state input; Stall_speed input; Wind_ned input; propulsion_data input; atmos_data input; data2 input; data3 input; data4 input; data5 input; data6 input; data7 input
function phi_d  = fcn(t, Thrust, mass, a_y_d,aero_data, structure_data,Plane_state,Stall_speed, Wind_ned, propulsion_data, atmos_data, data2, data3, data4, data5, data6, data7)
%%
b1=propulsion_data(1); % b and d of vtol propellers
d1=propulsion_data(2);
b1_inv=1.0/b1;
%%
rho=atmos_data(4); % density
%%

Tzf1=Thrust(1);
Tzf2=Thrust(2);
Tzf3=Thrust(3);
Tzf4=Thrust(4);

Tzb5=Thrust(5);
Tzb6=Thrust(6);
Tzb7=Thrust(7);
Tzb8=Thrust(8);
Tx9=Thrust(9);
Tx10=Thrust(10);
delta_e=Thrust(11);
delta_a=Thrust(12);
delta_r=Thrust(13);

TT=abs(Tzf1+Tzf2+Tzf3+Tzf4+Tzb5+Tzb6+Tzb7+Tzb8);

mass=structure_data(1,1);c=structure_data(1,2);b=structure_data(1,3);s=structure_data(1,4);
% Ix=structure_data(1,5);Iy=structure_data(1,6);Iz=structure_data(1,7);
% Ixy=structure_data(1,8);Ixz=structure_data(1,9);Iyz=structure_data(1,10);
% x1=structure_data(1,11);x2=structure_data(1,12);y1=structure_data(1,13);y2=structure_data(1,14);
% y3=structure_data(1,15);y4=structure_data(1,16);y5=structure_data(1,17);y6=structure_data(1,18);
% y7=structure_data(1,19);y8=structure_data(1,20);y9=structure_data(1,21);y10=structure_data(1,22);
% z1=structure_data(1,23);mb=structure_data(1,24);
% 
% T_by_W=2.0;

% c0=Ix*Iz-Ixz^2; 
% c1=Ixz*(Ix-Iy+Iz)/c0;    
% c2=(Iz*(Iz-Iy)+Ixz^2)/c0;                                              
% c3=Iz/c0;
% c4=Ixz/c0;
% c5=(Iz-Ix)/c0;
% c6=Ixz/Iy;
% c7=((Ix-Iy)*Ix + Ixz^2)/c0;
% c8=Ix/c0;
% c3_inv=1/c3;
% c8_inv=1/c8;

CLo =aero_data(1,1); CL_alpha=aero_data(1,2);CL_beta=aero_data(1,3); CL_delta_e=aero_data(1,4); CL_delta_a=aero_data(1,5); CL_delta_r=aero_data(1,6); CL_p=aero_data(1,7);CL_q=aero_data(1,8);CL_r=aero_data(1,9);

% Cdo =aero_data(1,1); Cd_alpha=aero_data(1,2);Cd_beta=aero_data(1,3); Cd_delta_e=aero_data(1,4); Cd_delta_a=aero_data(1,5); Cd_delta_r=aero_data(1,6); Cd_p=aero_data(1,7);Cd_q=aero_data(1,8);Cd_r=aero_data(1,9);
% 
% CYo =aero_data(1,1); CY_alpha=aero_data(1,2);CY_beta=aero_data(1,3); CY_delta_e=aero_data(1,4); CY_delta_a=aero_data(1,5); CY_delta_r=aero_data(1,6); CY_p=aero_data(1,7);CY_q=aero_data(1,8);CY_r=aero_data(1,9);
% 
% Clo =aero_data(1,1); Cl_alpha=aero_data(1,2);Cl_beta=aero_data(1,3); Cl_delta_e=aero_data(1,4); Cl_delta_a=aero_data(1,5); Cl_delta_r=aero_data(1,6); Cl_p=aero_data(1,7);Cl_q=aero_data(1,8);Cl_r=aero_data(1,9);
% 
% Cmo =aero_data(1,1); Cm_alpha=aero_data(1,2);Cm_beta=aero_data(1,3); Cm_delta_e=aero_data(1,4); Cm_delta_a=aero_data(1,5); Cm_delta_r=aero_data(1,6); Cm_p=aero_data(1,7);Cm_q=aero_data(1,8);Cm_r=aero_data(1,9);
% 
% Cno =aero_data(1,1); Cn_alpha=aero_data(1,2);Cn_beta=aero_data(1,3); Cn_delta_e=aero_data(1,4); Cn_delta_a=aero_data(1,5); Cn_delta_r=aero_data(1,6); Cn_p=aero_data(1,7);Cn_q=aero_data(1,8);Cn_r=aero_data(1,9);

% Cd_brake=0.0;brake=0.0;g=9.81;
% b1=0.0007488;
% d1=0.00002828;
% b1_inv=1.0/b1;

u=Plane_state(1);
v=Plane_state(2);
w=Plane_state(3);
 p=Plane_state(4);
 q=Plane_state(5);
 r=Plane_state(6);
phi=Plane_state(7);
theta=Plane_state(8);
psi=Plane_state(9);
% X=Plane_state(10);
% Y=Plane_state(11);
% Z=Plane_state(12);


R_v_v1=[cos(psi) sin(psi) 0; -sin(psi) cos(psi) 0; 0 0 1];
R_v1_v2=[cos(theta) 0 -sin(theta) ;0 1 0; sin(theta) 0 cos(theta)];
R_v2_b=[1 0 0;0 cos(phi) sin(phi) ;0 -sin(phi) cos(phi)];
R_v_b=R_v2_b*R_v1_v2*R_v_v1;



V_wind_bd=R_v_b*[Wind_ned(1);Wind_ned(2);Wind_ned(3)];

ppp = [u-V_wind_bd(1); v; w];
u_r=ppp(1);
v_r=ppp(2);
w_r=ppp(3);

V=sqrt(u_r^2+v_r^2+w_r^2);



if (u_r^2+v_r^2+w_r^2)<=0.01 
    alpha=0;
else
    alpha=atan2( w_r, u_r);
end

if norm(u_r) < 10^-3  && norm(v_r) < 10^-3 && norm(w_r) < 10^-3
    beta=0;
else
    beta = asin(v_r/sqrt(u_r^2+v_r^2+w_r^2));
end



R_b_s=[cos(alpha) 0 sin(alpha) ;0 1 0; -sin(alpha) 0 cos(alpha)]; 
R_s_w=[cos(beta) sin(beta) 0; -sin(beta) cos(beta) 0; 0 0 1];
R_w_b=(R_b_s)'*(R_s_w)';

% 
% mg_b = R_v_b*[0 ;0; mass*g];
% D=0.5*rho*V*V*s*(Cdo+Cd_alpha*abs(alpha)+Cd_delta_e*abs(delta_e)+ Cd_brake*abs(brake)) ;
% D_b=R_w_b*[-D;0;0];

if V<0.1
    CL = CLo + CL_alpha*alpha + CL_delta_e*delta_e ;
else
    CL = CLo + CL_alpha*alpha + CL_delta_e*delta_e  + CL_q*q*c/(2*V) ;
end

L=0.5*rho*V*V*s*(CL);
L_b = R_w_b*[0;0;-L];

if (abs(TT)<1)
    TT=1;
end
while (abs(mass*a_y_d/TT)) >= 0.7 %% 45 deg max
    TT=TT+1;
end

if (u_r<Stall_speed)
phi_d=asin((mass/TT)*a_y_d);
else
    phi_d=0.0;% R_circ= Inf
end

if abs(phi_d)>20/57.3
    phi_d = sign(phi_d)*20.0/57.3;
end

end

== matlab function Autopilot_q_full_5may_new/AUTOPILOT /Autopilot Transition mode/Reverse transition/Roll controller/MATLAB Function2 ==
  data: angular_state input; phi_dot_d input; p_d output
function p_d  = fcn(angular_state,phi_dot_d)
p=angular_state(1);
q=angular_state(2);
r=angular_state(3);
phi=angular_state(4);
theta=angular_state(5);
psi=angular_state(6);
p_d= phi_dot_d - q*sin(phi)*tan(theta)-r*cos(phi)*tan(theta);

end

== matlab function Autopilot_q_full_5may_new/AUTOPILOT /Autopilot Transition mode/Reverse transition/Heading Controller/MATLAB Function ==
  data: psi_d input; psi_error output; psi input
function psi_error = fcn(psi_d, psi)

psi_error=psi_d-psi;

if ( abs(psi_error) > pi )
    psi_error = -(psi_error/(abs(psi_error)))*abs((2*pi) - abs(psi_error));
end

end

== matlab function Autopilot_q_full_5may_new/AUTOPILOT /Autopilot Transition mode/Reverse transition/Heading Controller/MATLAB Function5 ==
  data: t input; psi_d output; u input; v input; psi_d input
function psi_d  = fcn(t,u,v, psi_d)


% if t>=35 && t<60
% psi_d= -(pi/50)*(t-35);
% end
% 
% 
% if t>=60 && t<85
%     psi_d= -(pi/2) - (pi/50)*(t-60);
% end
% 
% if t>=85 && t<110
%     psi_d= (pi) - (pi/50)*(t-85);
% end
% 
% if t>=110 && t<135
%     psi_d= (pi/2) - (pi/50)*(t-110);
% end
    
psi_d=psi_d;



end

== matlab function Autopilot_q_full_5may_new/AUTOPILOT /Autopilot Transition mode/Reverse transition/Heading Controller/MATLAB Function6 ==
  data: angular_state input; psi_dot_d input; r_d output
function r_d  = fcn(angular_state,psi_dot_d)

p=angular_state(1);
q=angular_state(2);
r=angular_state(3);
phi=angular_state(4);
theta=angular_state(5);
psi=angular_state(6);
if (abs(phi)>=((89.0)/57.3))
    phi=abs(phi)*89.0/(57.3*phi);
end

r_d = (psi_dot_d - q*sin(phi)*sec(theta))/(cos(phi)*sec(theta));
end
